simulink model "DFF_Block_Problem_Check"  (R2015b)
settings: Solver=VariableStepAuto  StartTime=0.0  StopTime=100.0  RelTol=1e-3
libraries: commutil2 x2, simulink x1, simulink_extras x1
settings Model: Creator=RamPrasadh  LastModifiedBy=RamPrasadh

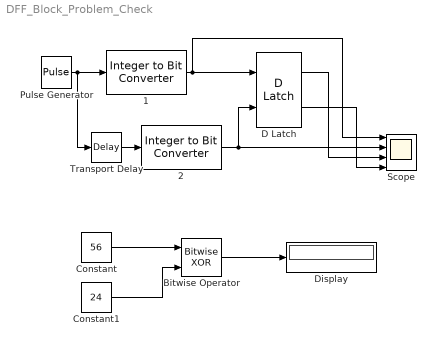
== system DFF_Block_Problem_Check ==
  "1 " : commutil2/Integer to Bit Converter  nbits=1  signedInputValues=Unsigned  bitOrder=MSB first  outDtype=boolean
  "2 " : commutil2/Integer to Bit Converter  nbits=1  signedInputValues=Unsigned  bitOrder=MSB first  outDtype=boolean
  Bitwise Operator : simulink/Logic and Bit Operations/Bitwise Operator  logicop=XOR  UseBitMask=off  NumInputPorts=2  BitMask=bin2dec('11011001')  BitMaskRealWorld=Stored Integer
  Constant : Constant  Value=56  OutDataTypeStr=uint8
  Constant1 : Constant  Value=24  OutDataTypeStr=uint8
  D Latch : simulink_extras/Flip Flops/D Latch
  Display : Display
  Pulse Generator : DiscretePulseGenerator  Period=7  PulseWidth=5  PhaseDelay=2
  Scope : Scope  NumInputPorts=4
  Transport Delay : TransportDelay  DelayTime=4
  wires:
  Pulse Generator/1 -> Transport Delay/1, "1 "/1
  Transport Delay/1 -> "2 "/1
  "1 "/1 -> D Latch/1, Scope/1
  "2 "/1 -> Scope/2, D Latch/2
  D Latch/1 -> Scope/3
  D Latch/2 -> Scope/4
  Constant/1 -> Bitwise Operator/1
  Constant1/1 -> Bitwise Operator/2
  Bitwise Operator/1 -> Display/1
